simulink model "EX003_FCHEV_simple"  (R2020b)
settings: Solver=ode23tb  StartTime=0.0  StopTime=20e3  MaxStep=1  RelTol=1e-3
libraries: component_lib x25, pid_lib x2
settings Model: Creator=maxjo65  LastModifiedBy=Max

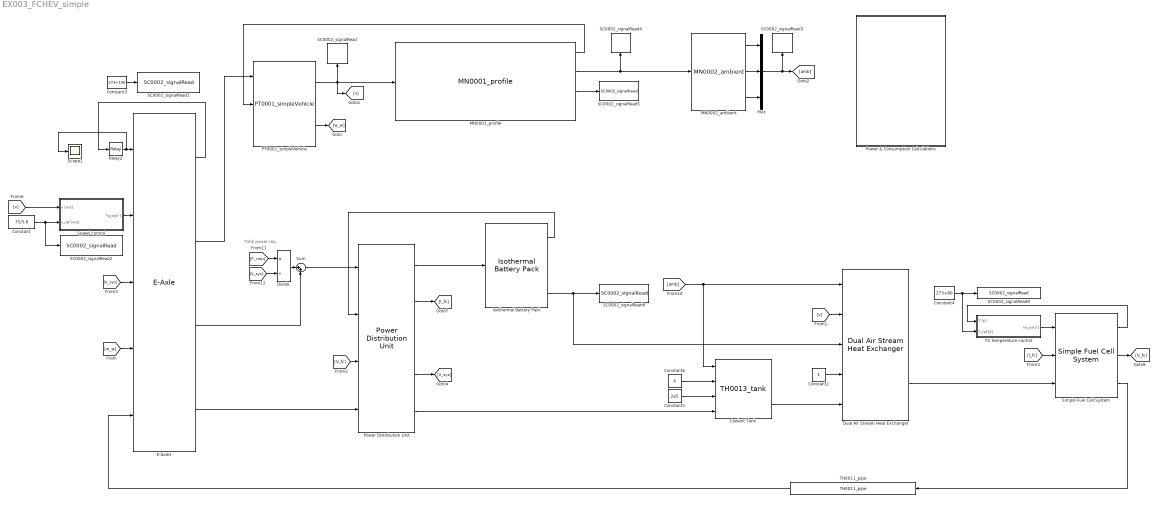
== system EX003_FCHEV_simple ==
  note: Total power req.
  Constant : Constant  Value=75/3.6
  Constant2 : Constant
  Constant3 : Constant  Value=273+100
  Constant4 : Constant  Value=273+80
  Constant5 : Constant  Value=2e5
  Constant6 : Constant  Value=4
  Coolant Tank : component_lib/Thermal Systems/TH0013_tank  V=5e-3
  Divide : Product  Inputs=*/
  Dual Air Stream Heat Exchanger : component_lib/Dual Air Stream Heat Exchanger  HtH=1.1  StS=0.95
  E-Axle1 : component_lib/E-Axle  n=2
  FC temperature control : Subsystem
  Isothermal Battery Pack : component_lib/Isothermal Battery Pack  SOC_0=0.5  n_mod_ser=16  n_mod_par=2  T=273+25
  MN0001_profile : component_lib/Mission/MN0001_profile  profile=Munchen.mat  x0=0  N_lookahead=100
  MN0002_ambient : component_lib/Mission/MN0002_ambient  p_0=1.01e5  T_0=273 + 20  RH_0=0.2
  Mux : Mux  Inputs=3
  PT0001_simpleVehicle : component_lib/Powertrain/PT0001_simpleVehicle  m=40e3  r_w=0.5  A_f=10  C_d=0.5  rho_air=1.225  c_r0=0.0060  c_r1=2.3e-7  gain=600  v0=75/3.6  x0=0
  Power & Consumption Calculations : Subsystem
  Power Distribution Unit : component_lib/Power Distribution Unit  V_sys=420  P_fc=150e3  I_bt_max=600  I_bt_min=-400  T_s=5
  Relay2 : Relay  OnSwitchValue=373+5  OffSwitchValue=373-5
  SC0002_signalRead : component_lib/Data & Control/SC0002_signalRead  SigName=velocity
  SC0002_signalRead1 : component_lib/Data & Control/SC0002_signalRead  SigName=motorTemperatureReference
  SC0002_signalRead2 : component_lib/Data & Control/SC0002_signalRead  SigName=velocityReference
  SC0002_signalRead3 : component_lib/Data & Control/SC0002_signalRead  SigName=ambient
  SC0002_signalRead4 : component_lib/Data & Control/SC0002_signalRead  SigName=altitude
  SC0002_signalRead5 : component_lib/Data & Control/SC0002_signalRead  SigName=distance
  SC0002_signalRead6 : component_lib/Data & Control/SC0002_signalRead  SigName=batteryHeatingPower
  SC0002_signalRead9 : component_lib/Data & Control/SC0002_signalRead  SigName=fuelCellTemperatureReference
  Scope1 : Scope
  Simple Fuel Cell System : component_lib/Simple Fuel Cell System  n_st=2
  Speed control : Subsystem
  Sum : Sum  Inputs=|++
  TH0011_pipe : component_lib/Thermal Systems/TH0011_pipe  d=3e-2  L=2  T_0=273 + 20  p_0=2e5  W_0=2
  wires:
  MN0001_profile/2 -> MN0002_ambient/1, SC0002_signalRead4/1
  Constant/1 -> Speed control/2(v_ref [m/s]), SC0002_signalRead2/1
  PT0001_simpleVehicle/1 -> SC0002_signalRead/1, [v], MN0001_profile/1
  PT0001_simpleVehicle/2 -> [w_w]
  MN0001_profile/1 -> PT0001_simpleVehicle/2
  [V_fc] -> Power Distribution Unit/3
  TH0011_pipe/1 -> E-Axle1/5
  Dual Air Stream Heat Exchanger/2 -> Simple Fuel Cell System/3
  Mux/1 -> [amb], SC0002_signalRead3/1
  [amb] -> Coolant Tank/1, Dual Air Stream Heat Exchanger/1
  MN0002_ambient/2 -> Mux/2
  MN0002_ambient/1 -> Mux/1
  MN0002_ambient/3 -> Mux/3
  Isothermal Battery Pack/1 -> Power Distribution Unit/2
  E-Axle1/4 -> Power Distribution Unit/4
  Power Distribution Unit/2 -> [I_fc]
  Power Distribution Unit/4 -> [V_sys]
  Power Distribution Unit/5 -> Coolant Tank/4
  MN0001_profile/3 -> SC0002_signalRead5/1
  Coolant Tank/2 -> Dual Air Stream Heat Exchanger/5
  Constant5/1 -> Coolant Tank/3
  Constant6/1 -> Coolant Tank/2
  Constant4/1 -> FC temperature control/2(T_ref [K]), SC0002_signalRead9/1
  Power Distribution Unit/1 -> Isothermal Battery Pack/1
  [V_sys] -> E-Axle1/3
  [w_w] -> E-Axle1/4
  Speed control/1(Tq_sig [-]) -> E-Axle1/2
  E-Axle1/2 -> PT0001_simpleVehicle/1
  [v] -> Speed control/1(v [m/s])
  Constant3/1 -> SC0002_signalRead1/1
  Relay2/1 -> Scope1/1, E-Axle1/1
  E-Axle1/1 -> Relay2/1
  [v] -> Dual Air Stream Heat Exchanger/2
  Simple Fuel Cell System/3 -> TH0011_pipe/1
  Simple Fuel Cell System/2 -> [V_fc]
  FC temperature control/1(th_ctrl [-]) -> Simple Fuel Cell System/1
  Simple Fuel Cell System/1 -> FC temperature control/1(T [K])
  Sum/1 -> Power Distribution Unit/1
  [P_cmp] -> Divide/1
  [V_sys] -> Divide/2
  Divide/1 -> Sum/1
  E-Axle1/3 -> Sum/2
  Constant2/1 -> Dual Air Stream Heat Exchanger/4
  Isothermal Battery Pack/3 -> Dual Air Stream Heat Exchanger/3, SC0002_signalRead6/1
  [I_fc] -> Simple Fuel Cell System/2

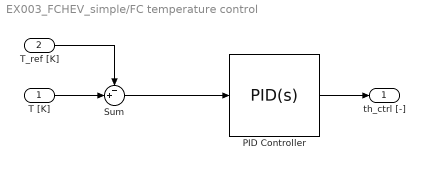
== system EX003_FCHEV_simple/FC temperature control ==
  T [K] : Inport
  T_ref [K] : Inport  Port=2
  PID Controller : pid_lib/PID Controller  Controller=PID  Form=Parallel  TimeDomain=Continuous-time  UseExternalTs=off  SampleTime=-1  IntegratorMethod=Forward Euler  FilterMethod=Forward Euler  ControllerParametersSource=internal  P=1e-2  I=1e-3  D=0  UseFilter=on  N=100  TunerSelectOption=Transfer Function Based (PID Tuner App)  InitialConditionSource=internal  InitialConditionForIntegrator=0  InitialConditionForFilter=0  DifferentiatorICPrevScaledInput=0  ExternalReset=none  TrackingMode=off  Kt=1  LimitOutput=on  SatLimitsSource=internal  UpperSaturationLimit=1  LowerSaturationLimit=0  LinearizeAsGain=on  AntiWindupMode=clamping  Kb=1  POutMin=[]  POutMax=[]  IOutMin=[]  IOutMax=[]  DOutMin=[]  DOutMax=[]  NOutMin=[]  NOutMax=[]  SumOutMin=[]  SumOutMax=[]  SaturationOutMin=[]  SaturationOutMax=[]  PParamMin=[]  PParamMax=[]  IParamMin=[]  IParamMax=[]  DParamMin=[]  DParamMax=[]  NParamMin=[]  NParamMax=[]  KbParamMin=[]  KbParamMax=[]  KtParamMin=[]  KtParamMax=[]  KbOutMin=[]  KbOutMax=[]  KtOutMin=[]  KtOutMax=[]  IntegratorOutMin=[]  IntegratorOutMax=[]  FilterOutMin=[]  FilterOutMax=[]  SumI1OutMin=[]  SumI1OutMax=[]  SumI2OutMin=[]  SumI2OutMax=[]  SumI3OutMin=[]  SumI3OutMax=[]  SumI4OutMin=[]  SumI4OutMax=[]  SumDOutMin=[]  SumDOutMax=[]  DifferentiatorOutMin=[]  DifferentiatorOutMax=[]  FilterDiffOutCoefMin=[]  FilterDiffOutCoefMax=[]  ReciprocalOutMin=[]  ReciprocalOutMax=[]  SumDenOutMin=[]  SumDenOutMax=[]  SumNumOutMin=[]  SumNumOutMax=[]  DivideOutMin=[]  DivideOutMax=[]  UdiffTsProdOutMin=[]  UdiffTsProdOutMax=[]  NTsProdOutMin=[]  NTsProdOutMax=[]  UintegralTsProdOutMin=[]  UintegralTsProdOutMax=[]  UngainTsProdOutMin=[]  UngainTsProdOutMax=[]  IntegratorContinuousStateAttributes=''  IntegratorStateMustResolveToSignalObject=off  IntegratorRTWStateStorageClass=Auto  FilterContinuousStateAttributes=''  FilterStateMustResolveToSignalObject=off  FilterRTWStateStorageClass=Auto  ParallelPVariant=InternalParameters  IdealPVariant=Disabled  IVariant=InternalParameters  DVariant=InternalParameters  IntegratorVariant=Continuous  SatVariant=Enabled  AWVariant=ContClampingParallel  PCopyVariant=Disabled  TRVariant=Disabled  FdbkBlocksVariant=Forward  IdealPFdbkVariant=Disabled  SatFdbkVariant=Disabled  DerivativeFilterVariant=ContFilter  NVariant=InternalParameters  NCopyVariant=Disabled  FilterICVariant=InternalICsFilter  IntegratorICVariant=InternalICs  ExternalResetVariant=Disabled  TRSumVariant=Passthrough  SumFdbkVariant=Disabled  SumVariant=Sum_PID  TsampFilterVariant=InternalTs  TsampNgainVariant=Passthrough  TsampIntegralVariant=Passthrough  ExternalSaturationOutDataTypeStr=Inherit: Same as second input
  Sum : Sum  Inputs=-+|
  th_ctrl [-] : Outport
  wires:
  PID Controller/1 -> th_ctrl [-]/1
  T_ref [K]/1 -> Sum/1
  T [K]/1 -> Sum/2
  Sum/1 -> PID Controller/1

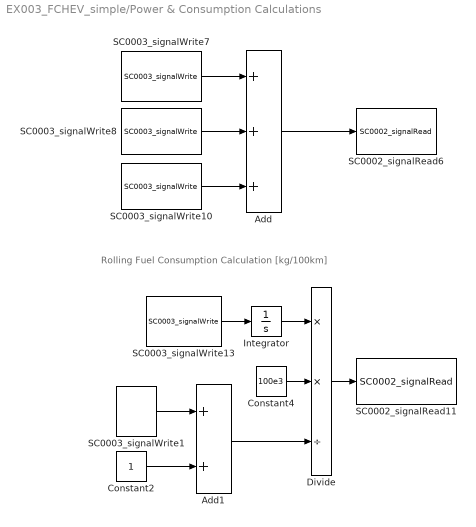
== system EX003_FCHEV_simple/Power & Consumption Calculations ==
  note: Rolling Fuel Consumption Calculation [kg/100km]
  Add : Sum  Inputs=+++
  Add1 : Sum
  Constant2 : Constant
  Constant4 : Constant  Value=100e3
  Divide : Product  Inputs=**/
  Integrator : Integrator
  SC0002_signalRead11 : component_lib/Data & Control/SC0002_signalRead  SigName=fuelConsumption
  SC0002_signalRead6 : component_lib/Data & Control/SC0002_signalRead  SigName=producedPower
  SC0003_signalWrite1 : component_lib/Data & Control/SC0003_signalWrite  SigName=distance
  SC0003_signalWrite10 : component_lib/Data & Control/SC0003_signalWrite  SigName=burnOffPower
  SC0003_signalWrite13 : component_lib/Data & Control/SC0003_signalWrite  SigName=hydrogenFlow
  SC0003_signalWrite7 : component_lib/Data & Control/SC0003_signalWrite  SigName=batteryPower
  SC0003_signalWrite8 : component_lib/Data & Control/SC0003_signalWrite  SigName=fuelCellPower
  wires:
  Integrator/1 -> Divide/1
  SC0003_signalWrite7/1 -> Add/1
  SC0003_signalWrite10/1 -> Add/3
  SC0003_signalWrite1/1 -> Add1/1
  SC0003_signalWrite8/1 -> Add/2
  Add/1 -> SC0002_signalRead6/1
  Add1/1 -> Divide/3
  Constant4/1 -> Divide/2
  Constant2/1 -> Add1/2
  Divide/1 -> SC0002_signalRead11/1
  SC0003_signalWrite13/1 -> Integrator/1

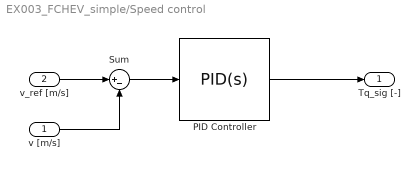
== system EX003_FCHEV_simple/Speed control ==
  v [m/s] : Inport
  v_ref [m/s] : Inport  Port=2
  PID Controller : pid_lib/PID Controller  Controller=PID  Form=Parallel  TimeDomain=Continuous-time  UseExternalTs=off  SampleTime=-1  IntegratorMethod=Forward Euler  FilterMethod=Forward Euler  ControllerParametersSource=internal  P=10  I=1e-1  D=0  UseFilter=on  N=100  TunerSelectOption=Transfer Function Based (PID Tuner App)  InitialConditionSource=internal  InitialConditionForIntegrator=0  InitialConditionForFilter=0  DifferentiatorICPrevScaledInput=0  ExternalReset=none  TrackingMode=off  Kt=1  LimitOutput=on  SatLimitsSource=internal  UpperSaturationLimit=1  LowerSaturationLimit=-1  LinearizeAsGain=on  AntiWindupMode=clamping  Kb=1  POutMin=[]  POutMax=[]  IOutMin=[]  IOutMax=[]  DOutMin=[]  DOutMax=[]  NOutMin=[]  NOutMax=[]  SumOutMin=[]  SumOutMax=[]  SaturationOutMin=[]  SaturationOutMax=[]  PParamMin=[]  PParamMax=[]  IParamMin=[]  IParamMax=[]  DParamMin=[]  DParamMax=[]  NParamMin=[]  NParamMax=[]  KbParamMin=[]  KbParamMax=[]  KtParamMin=[]  KtParamMax=[]  KbOutMin=[]  KbOutMax=[]  KtOutMin=[]  KtOutMax=[]  IntegratorOutMin=[]  IntegratorOutMax=[]  FilterOutMin=[]  FilterOutMax=[]  SumI1OutMin=[]  SumI1OutMax=[]  SumI2OutMin=[]  SumI2OutMax=[]  SumI3OutMin=[]  SumI3OutMax=[]  SumI4OutMin=[]  SumI4OutMax=[]  SumDOutMin=[]  SumDOutMax=[]  DifferentiatorOutMin=[]  DifferentiatorOutMax=[]  FilterDiffOutCoefMin=[]  FilterDiffOutCoefMax=[]  ReciprocalOutMin=[]  ReciprocalOutMax=[]  SumDenOutMin=[]  SumDenOutMax=[]  SumNumOutMin=[]  SumNumOutMax=[]  DivideOutMin=[]  DivideOutMax=[]  UdiffTsProdOutMin=[]  UdiffTsProdOutMax=[]  NTsProdOutMin=[]  NTsProdOutMax=[]  UintegralTsProdOutMin=[]  UintegralTsProdOutMax=[]  UngainTsProdOutMin=[]  UngainTsProdOutMax=[]  IntegratorContinuousStateAttributes=''  IntegratorStateMustResolveToSignalObject=off  IntegratorRTWStateStorageClass=Auto  FilterContinuousStateAttributes=''  FilterStateMustResolveToSignalObject=off  FilterRTWStateStorageClass=Auto  ParallelPVariant=InternalParameters  IdealPVariant=Disabled  IVariant=InternalParameters  DVariant=InternalParameters  IntegratorVariant=Continuous  SatVariant=Enabled  AWVariant=ContClampingParallel  PCopyVariant=Disabled  TRVariant=Disabled  FdbkBlocksVariant=Forward  IdealPFdbkVariant=Disabled  SatFdbkVariant=Disabled  DerivativeFilterVariant=ContFilter  NVariant=InternalParameters  NCopyVariant=Disabled  FilterICVariant=InternalICsFilter  IntegratorICVariant=InternalICs  ExternalResetVariant=Disabled  TRSumVariant=Passthrough  SumFdbkVariant=Disabled  SumVariant=Sum_PID  TsampFilterVariant=InternalTs  TsampNgainVariant=Passthrough  TsampIntegralVariant=Passthrough  ExternalSaturationOutDataTypeStr=Inherit: Same as second input
  Sum : Sum  Inputs=|+-
  Tq_sig [-] : Outport
  wires:
  PID Controller/1 -> Tq_sig [-]/1
  Sum/1 -> PID Controller/1
  v_ref [m/s]/1 -> Sum/1
  v [m/s]/1 -> Sum/2
